simulink model "solar_thermal_control"  (R2024a)
settings: Solver=VariableStepAuto  StartTime=0.0  StopTime=3600*24  FixedStep=0.01  RelTol=1e-3
libraries: fl_lib x41, nesl_utility x20, SimscapeFluids_lib x1
settings Model: Creator=fanzh  LastModifiedBy=fanzh

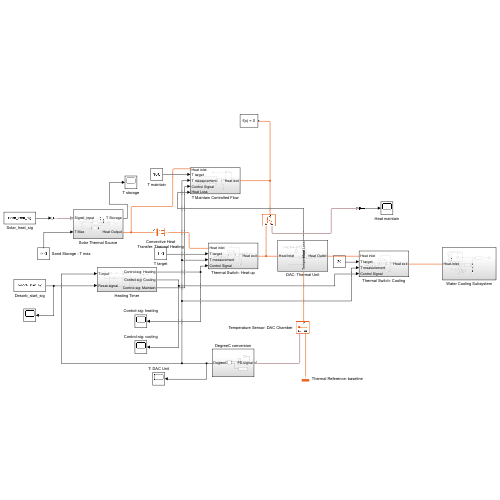
[thumbnail: Simulink's stored preview of the top-level diagram]
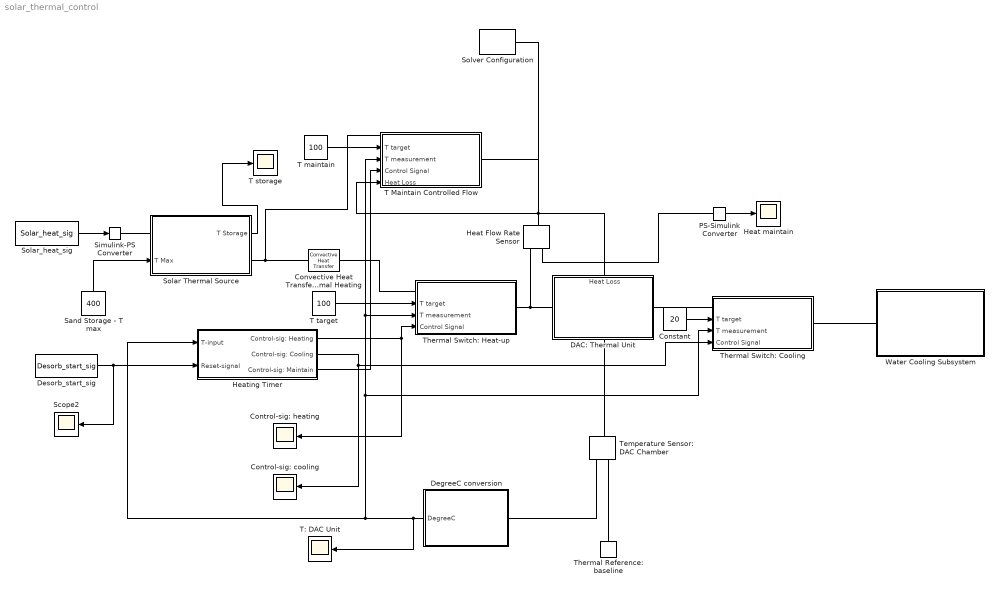
== system solar_thermal_control ==
  Constant : Constant  Value=20
  Control-sig: cooling : Scope
  Control-sig: heating : Scope
  Convective Heat Transfer: Thermal Heating : fl_lib/Thermal/Thermal Elements/Convective Heat Transfer  thermal_type=foundation.enum.constant_variable.constant  area=0.1 m^2  heat_tr_coeff=150 W/(K*m^2)  min_heat_tr_coeff=1e-3 W/(K*m^2)  T_specify=off  T_priority=None  T=0 K  T_nominal_specify=off  T_nominal_value=1  T_nominal_unit=K  Q_specify=off  Q_priority=None  Q=0 W  Q_nominal_specify=off  Q_nominal_value=1  Q_nominal_unit=W
  DAC: Thermal Unit : Subsystem
      settings: PortSchema="{\"entries\":[{\"content\":{\"sides\":[{\"content\":{\"connectorIds\":[\"LConn1\"]},\"type\":\"ConnectorPlacement.EquallySpacedRectSide\",\"uuid\":\"21b9ae42-c24c-4450-b3a3-af5fe19a1042\"},{\"content\":{\"connectorIds\":[\"RConn1\"],\"side\":\"RIGHT\"},\"type\":\"ConnectorPlacement.EquallySpacedRectSide\",\"uuid\":\"0b7693d4-30f7-45cc-b119-858b172421da\"},{\"content\":{\"connectorIds\":[\"Out1\"],\"side\":\"TOP\"},\"type\":\"ConnectorPlacement.EquallySpacedRectSide\",\"uuid\":\"dc3a2d3c-c181-42f7-acd1-46fa5c20e34e\"},{\"content\":{\"connectorIds\":[\"RConn2\"],\"side\":\"BOTTOM\"},\"type\":\"ConnectorPlacement.EquallySpacedRectSide\",\"uuid\":\"1fa3cf11-aa97-4b08-a978-f3583bb285c7\"}]},\"type\":\"ConnectorPlacement.EquallySpacedConnector\",\"uuid\":\"5312b09c-b763-4a63-a4e3-3dc47fafb726\"}],\"packageUris\":[\"http://schema.mathworks.com/mf0/Connector/R2020b\"],\"version\":\"1.0\"}"
  DegreeC conversion : Subsystem
  Desorb_start_sig : FromWorkspace  VariableName=Desorb_start_sig  OutDataTypeStr=boolean  SampleTime=10  Interpolate=off  ZeroCross=off  OutputAfterFinalValue=Holding final value
  Heat Flow Rate Sensor : fl_lib/Thermal/Thermal Sensors/Heat Flow Rate Sensor
  Heat maintain : Scope
  Heating Timer : Subsystem
  PS-Simulink Converter : nesl_utility/PS-Simulink Converter  PhysicalDomain=network_engine_domain  SubClassName=ps_output  LeftPortType=input  RightPortType=output  PseudoPeriodic=off  Frequencies=[]  VectorFormat=inherit  Unit=inherit  AffineConversion=off
  Sand Storage - T max : Constant  Value=400
  Scope2 : Scope
  Simulink-PS Converter : nesl_utility/Simulink-PS Converter  PhysicalDomain=network_engine_domain  SubClassName=ps_input  LeftPortType=input  RightPortType=output  PseudoPeriodic=off  Frequencies=[]  NoiseDistribution=none  NoiseParameters=[]  Unit=J/s  AffineConversion=off  FilteringAndDerivatives=provide  SimscapeFilterOrder=1  InputFilterTimeConstant=0.001  UdotUserProvided=0
  Solar Thermal Source : Subsystem
      settings: PortSchema="{\"entries\":[{\"content\":{\"sides\":[{\"content\":{\"connectorIds\":[\"LConn1\",\"In1\"]},\"type\":\"ConnectorPlacement.EquallySpacedRectSide\",\"uuid\":\"f69a8d61-d6b7-4c5f-bee5-6777f6738a93\"},{\"content\":{\"connectorIds\":[\"Out1\",\"RConn1\"],\"side\":\"RIGHT\"},\"type\":\"ConnectorPlacement.EquallySpacedRectSide\",\"uuid\":\"2abf6aad-3ae7-4bac-8cd7-a5726210c2fc\"},{\"content\":{\"side\":\"TOP\"},\"type\":\"ConnectorPlacement.EquallySpacedRectSide\",\"uuid\":\"e643bfa7-5cdc-456c-a6d6-e9bc07f127d5\"}]},\"type\":\"ConnectorPlacement.EquallySpacedConnector\",\"uuid\":\"a763efd1-4c7b-49c2-88ea-f9b1ada0c58b\"}],\"packageUris\":[\"http://schema.mathworks.com/mf0/Connector/R2020b\"],\"version\":\"1.0\"}"
  Solar_heat_sig : FromWorkspace  VariableName=Solar_heat_sig  SampleTime=10  Interpolate=off  ZeroCross=off  OutputAfterFinalValue=Holding final value
  Solver Configuration : nesl_utility/Solver Configuration  PhysicalDomain=network_engine_domain  SubClassName=solver  LeftPortType=input  RightPortType=generic  Tones=[]  Harmonics=[]  SimulateNoise=off  Profile=off  UseLocalSampling=off  EnableSwitchedLinearOptims=on  FrequencyDomain=off  UseCCode=off  RelTol=0.001  AbsTol=0.001  MinStep=1e-09  ToWorkspace=off  RevertToSquareIcSolve=off  NumHomotopyIterations=100  PhasorMode=off  PhasorModeNumHarmonics=1  ConsistencySolver=NEWTON_XTOL_AFTER_FTOL  IndexReductionMethod=DerivativeReplacement  DoDC=off  ResidualTolerance=1e-09  ConsistencyTolSource=GLOBAL  ConsistencyAbsTol=0.001  ConsistencyRelTol=0.001  ConsistencyTolFactor=0.001  UseLocalSolver=off  LocalSolverChoice=NE_BACKWARD_EULER_ADVANCER  ResolveIndetEquations=on  FunctionEvalNumThread=1  LocalSolverSampleTime=0.001  DoFixedCost=off  MaxNonlinIter=3  MaxModeIter=2  ComputeImpulses=off  ImpulseIterations=2  LinearAlgebra=auto  LinearAlgebraNumThread=0  EquationFormulation=NE_TIME_EF  DelaysMemoryBudget=1024  AutomaticFiltering=on  FilteringTimeConstant=0.001  PartitionStorageMethod=AS_NEEDED  PartitionMemoryBudget=1024  PartitionMethod=ROBUST  MultibodyUseLocalSolver=off  MultibodyLocalSolverChoice=ODE1  MultibodyLocalSolverSampleTime=0.001
  T Maintain Controlled Flow : Subsystem
      settings: PortSchema="{\"entries\":[{\"content\":{\"sides\":[{\"content\":{\"connectorIds\":[\"LConn1\",\"In1\",\"In2\",\"In3\",\"In4\"]},\"type\":\"ConnectorPlacement.EquallySpacedRectSide\",\"uuid\":\"eab90983-c678-4d00-88f4-d7eb0332fabb\"},{\"content\":{\"connectorIds\":[\"RConn1\"],\"side\":\"RIGHT\"},\"type\":\"ConnectorPlacement.EquallySpacedRectSide\",\"uuid\":\"4911cae5-9d9f-472e-86e2-92bac9c7b6a6\"},{\"content\":{\"side\":\"TOP\"},\"type\":\"ConnectorPlacement.EquallySpacedRectSide\",\"uuid\":\"e0869e9b-2d53-4209-96a5-637bff90aadc\"}]},\"type\":\"ConnectorPlacement.EquallySpacedConnector\",\"uuid\":\"c03f20a9-89c5-4bd4-ab09-4122887b8deb\"}],\"packageUris\":[\"http://schema.mathworks.com/mf0/Connector/R2020b\"],\"version\":\"1.0\"}"
  T maintain : Constant  Value=100
  T storage : Scope
  T target : Constant  Value=100
  T: DAC Unit : Scope
  "Temperature Sensor: DAC Chamber " : fl_lib/Thermal/Thermal Sensors/Temperature Sensor  temperature_measure=foundation.enum.MeasurementReference.difference
  Thermal Reference: baseline : fl_lib/Thermal/Thermal Elements/Thermal Reference
  Thermal Switch: Cooling : Subsystem
      settings: PortSchema="{\"entries\":[{\"content\":{\"sides\":[{\"content\":{\"connectorIds\":[\"LConn1\",\"In1\",\"In2\",\"In3\"]},\"type\":\"ConnectorPlacement.EquallySpacedRectSide\",\"uuid\":\"eab90983-c678-4d00-88f4-d7eb0332fabb\"},{\"content\":{\"connectorIds\":[\"RConn1\"],\"side\":\"RIGHT\"},\"type\":\"ConnectorPlacement.EquallySpacedRectSide\",\"uuid\":\"4911cae5-9d9f-472e-86e2-92bac9c7b6a6\"},{\"content\":{\"side\":\"TOP\"},\"type\":\"ConnectorPlacement.EquallySpacedRectSide\",\"uuid\":\"e0869e9b-2d53-4209-96a5-637bff90aadc\"}]},\"type\":\"ConnectorPlacement.EquallySpacedConnector\",\"uuid\":\"c03f20a9-89c5-4bd4-ab09-4122887b8deb\"}],\"packageUris\":[\"http://schema.mathworks.com/mf0/Connector/R2020b\"],\"version\":\"1.0\"}"
  Thermal Switch: Heat-up : Subsystem
      settings: PortSchema="{\"entries\":[{\"content\":{\"sides\":[{\"content\":{\"connectorIds\":[\"LConn1\",\"In1\",\"In2\",\"In3\"]},\"type\":\"ConnectorPlacement.EquallySpacedRectSide\",\"uuid\":\"eab90983-c678-4d00-88f4-d7eb0332fabb\"},{\"content\":{\"connectorIds\":[\"RConn1\"],\"side\":\"RIGHT\"},\"type\":\"ConnectorPlacement.EquallySpacedRectSide\",\"uuid\":\"4911cae5-9d9f-472e-86e2-92bac9c7b6a6\"},{\"content\":{\"side\":\"TOP\"},\"type\":\"ConnectorPlacement.EquallySpacedRectSide\",\"uuid\":\"e0869e9b-2d53-4209-96a5-637bff90aadc\"}]},\"type\":\"ConnectorPlacement.EquallySpacedConnector\",\"uuid\":\"c03f20a9-89c5-4bd4-ab09-4122887b8deb\"}],\"packageUris\":[\"http://schema.mathworks.com/mf0/Connector/R2020b\"],\"version\":\"1.0\"}"
  Water Cooling Subsystem : Subsystem
  wires:
  T target/1 -> Thermal Switch: Heat-up/1(T target)
  Constant/1 -> Thermal Switch: Cooling/1(T target)
  Heating Timer/1(Control-sig: Heating) -> Control-sig: heating/1, Thermal Switch: Heat-up/3(Control Signal)
  Heating Timer/2(Control-sig: Cooling) -> Control-sig: cooling/1, Thermal Switch: Cooling/3(Control Signal)
  Solar_heat_sig/1 -> Simulink-PS Converter/1
  Sand Storage - T max/1 -> Solar Thermal Source/1(T Max)
  Desorb_start_sig/1 -> Heating Timer/2(Reset-signal), Scope2/1
  T maintain/1 -> T Maintain Controlled Flow/1(T target)
  PS-Simulink Converter/1 -> Heat maintain/1
  Heating Timer/3(Control-sig: Maintain) -> T Maintain Controlled Flow/3(Control Signal)
  DegreeC conversion/1(DegreeC) -> Thermal Switch: Cooling/2(T measurement), Thermal Switch: Heat-up/2(T measurement), T Maintain Controlled Flow/2(T measurement), Heating Timer/1(T-input), T: DAC Unit/1
  Solar Thermal Source/1(T Storage) -> T storage/1
  DAC: Thermal Unit/1(Heat Loss) -> T Maintain Controlled Flow/4(Heat Loss)
  connections:
  "Temperature Sensor: DAC Chamber "/RConn1 -- Thermal Reference: baseline/LConn1
  Thermal Switch: Heat-up/RConn1 -- Heat Flow Rate Sensor/RConn2 -- DAC: Thermal Unit/LConn1
  Thermal Switch: Heat-up/LConn1 -- Convective Heat Transfer: Thermal Heating/RConn1
  "Temperature Sensor: DAC Chamber "/LConn1 -- DAC: Thermal Unit/RConn2
  "Temperature Sensor: DAC Chamber "/RConn2 -- DegreeC conversion/LConn1
  DAC: Thermal Unit/RConn1 -- Thermal Switch: Cooling/LConn1
  Water Cooling Subsystem/LConn1 -- Thermal Switch: Cooling/RConn1
  Simulink-PS Converter/RConn1 -- Solar Thermal Source/LConn1
  PS-Simulink Converter/LConn1 -- Heat Flow Rate Sensor/RConn1
  Heat Flow Rate Sensor/LConn1 -- T Maintain Controlled Flow/RConn1 -- Solver Configuration/RConn1
  Convective Heat Transfer: Thermal Heating/LConn1 -- T Maintain Controlled Flow/LConn1 -- Solar Thermal Source/RConn1

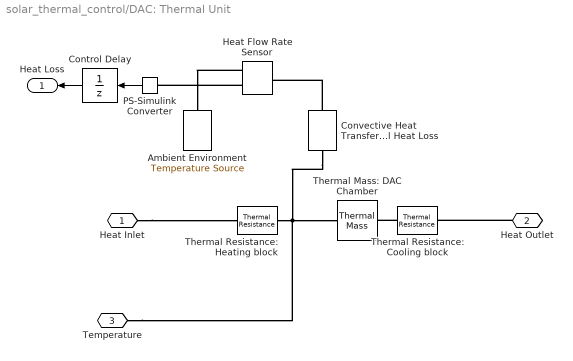
== system solar_thermal_control/DAC: Thermal Unit ==
  Ambient Environment : fl_lib/Thermal/Thermal Sources/Temperature Source  temperature=15 degC
  Control Delay : UnitDelay  SampleTime=-1  HasFrameUpgradeWarning=on
  Convective Heat Transfer: Natural Heat Loss : fl_lib/Thermal/Thermal Elements/Convective Heat Transfer  thermal_type=foundation.enum.constant_variable.constant  area=0.05 m^2  heat_tr_coeff=4 W/(K*m^2)  min_heat_tr_coeff=1e-3 W/(K*m^2)  T_specify=off  T_priority=None  T=0 K  T_nominal_specify=off  T_nominal_value=1  T_nominal_unit=K  Q_specify=off  Q_priority=None  Q=0 W  Q_nominal_specify=off  Q_nominal_value=1  Q_nominal_unit=W
  Heat Flow Rate Sensor : fl_lib/Thermal/Thermal Sensors/Heat Flow Rate Sensor
  PS-Simulink Converter : nesl_utility/PS-Simulink Converter  PhysicalDomain=network_engine_domain  SubClassName=ps_output  LeftPortType=input  RightPortType=output  PseudoPeriodic=off  Frequencies=[]  VectorFormat=inherit  Unit=inherit  AffineConversion=off
  Thermal Mass: DAC Chamber : fl_lib/Thermal/Thermal Elements/Thermal Mass  mass_type=foundation.enum.constant_variable.constant  mass=2 kg  sp_heat=447 J/(K*kg)  mass_min=1e-6 kg  num_ports=foundation.enum.numPorts2.two  m_specify=off  m_priority=High  m=1 kg  m_nominal_specify=off  m_nominal_value=1  m_nominal_unit=kg  T_specify=on  T_priority=High  T=15 degC  T_nominal_specify=off  T_nominal_value=1  T_nominal_unit=K  Q_specify=off  Q_priority=None  Q=0 W  Q_nominal_specify=off  Q_nominal_value=1  Q_nominal_unit=W
      settings: InternalSimscapePortConfiguration="{\"Bottom\":[],\"Left\":[{\"id\":\"M\",\"label\":\"\",\"type\":\"foundation.thermal.thermal\"}],\"Right\":[{\"id\":\"N\",\"label\":\"\",\"type\":\"foundation.thermal.thermal\"}],\"Top\":[]}"
  Thermal Resistance: Cooling block : fl_lib/Thermal/Thermal Elements/Thermal Resistance  resistance=0.1 K/W  T_specify=off  T_priority=None  T=0 K  T_nominal_specify=off  T_nominal_value=1  T_nominal_unit=K  Q_specify=off  Q_priority=None  Q=0 W  Q_nominal_specify=off  Q_nominal_value=1  Q_nominal_unit=W
  Thermal Resistance: Heating block : fl_lib/Thermal/Thermal Elements/Thermal Resistance  resistance=1 K/W  T_specify=off  T_priority=None  T=0 K  T_nominal_specify=off  T_nominal_value=1  T_nominal_unit=K  Q_specify=off  Q_priority=None  Q=0 W  Q_nominal_specify=off  Q_nominal_value=1  Q_nominal_unit=W
  Heat Inlet : PMIOPort  Side=Left
  Heat Outlet : PMIOPort  Port=2  Side=Right
  Temperature : PMIOPort  Port=3  Side=Right
  Heat Loss : Outport
  wires:
  PS-Simulink Converter/1 -> Control Delay/1
  Control Delay/1 -> Heat Loss/1
  connections:
  Heat Inlet/RConn1 -- Thermal Resistance: Heating block/LConn1
  Thermal Resistance: Heating block/RConn1 -- Thermal Mass: DAC Chamber/LConn1 -- Convective Heat Transfer: Natural Heat Loss/LConn1 -- Temperature/RConn1
  Thermal Resistance: Cooling block/LConn1 -- Thermal Mass: DAC Chamber/RConn1
  Heat Outlet/RConn1 -- Thermal Resistance: Cooling block/RConn1
  Convective Heat Transfer: Natural Heat Loss/RConn1 -- Heat Flow Rate Sensor/LConn1
  Heat Flow Rate Sensor/RConn2 -- Ambient Environment/LConn1
  Heat Flow Rate Sensor/RConn1 -- PS-Simulink Converter/LConn1

== system solar_thermal_control/DegreeC conversion ==
  Absolute zero reference : Constant  Value=-273.15
  PS-Simulink Converter : nesl_utility/PS-Simulink Converter  PhysicalDomain=network_engine_domain  SubClassName=ps_output  LeftPortType=input  RightPortType=output  PseudoPeriodic=off  Frequencies=[]  VectorFormat=inherit  Unit=inherit  AffineConversion=off
  T: degreeC : Sum
  PS-signal : PMIOPort  Side=Left
  DegreeC : Outport
  wires:
  Absolute zero reference/1 -> T: degreeC/2
  PS-Simulink Converter/1 -> T: degreeC/1
  T: degreeC/1 -> DegreeC/1
  connections:
  PS-signal/RConn1 -- PS-Simulink Converter/LConn1

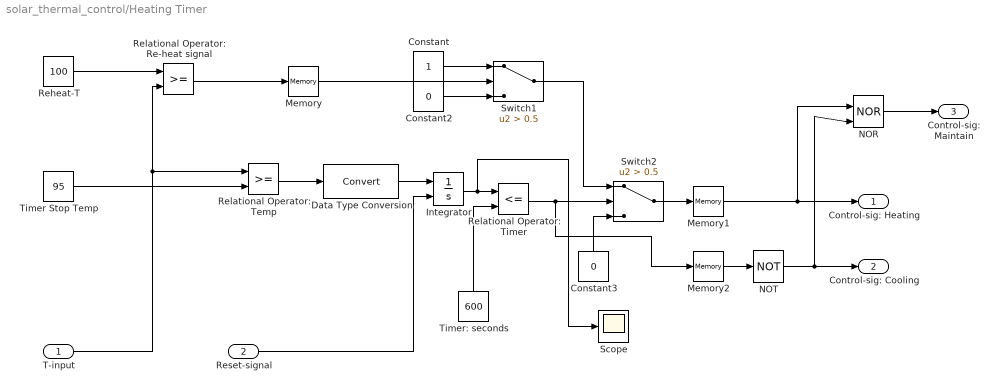
== system solar_thermal_control/Heating Timer ==
  T-input : Inport
  Reset-signal : Inport  Port=2
  Constant : Constant
  Constant2 : Constant  Value=0
  Constant3 : Constant  Value=0
  Data Type Conversion : DataTypeConversion  SaturateOnIntegerOverflow=off  RndMeth=Floor
  Integrator : Integrator  ExternalReset=level hold
  Memory : Memory
  Memory1 : Memory
  Memory2 : Memory
  NOR : Logic  Operator=NOR  IconShape=distinctive  AllPortsSameDT=off  OutDataTypeStr=boolean
  NOT : Logic  Operator=NOT  IconShape=distinctive  AllPortsSameDT=off  OutDataTypeStr=boolean
  Reheat-T : Constant  Value=100
  Relational Operator: Re-heat signal : RelationalOperator  OutDataTypeStr=boolean  RndMeth=Simplest  InputSameDT=off
  Relational Operator: Temp : RelationalOperator  OutDataTypeStr=boolean  RndMeth=Simplest  InputSameDT=off
  Relational Operator: Timer : RelationalOperator  Operator=<=  OutDataTypeStr=boolean  RndMeth=Simplest  InputSameDT=off
  Scope : Scope
  Switch1 : Switch  Criteria=u2 > Threshold  Threshold=0.5  SaturateOnIntegerOverflow=off  InputSameDT=off
  Switch2 : Switch  Criteria=u2 > Threshold  Threshold=0.5  SaturateOnIntegerOverflow=off  InputSameDT=off
  Timer Stop Temp : Constant  Value=95
  Timer: seconds : Constant  Value=600
  Control-sig: Heating : Outport
  Control-sig: Cooling : Outport  Port=2
  Control-sig: Maintain : Outport  Port=3
  wires:
  Relational Operator: Temp/1 -> Data Type Conversion/1
  T-input/1 -> Relational Operator: Re-heat signal/2, Relational Operator: Temp/1
  Data Type Conversion/1 -> Integrator/1
  Timer Stop Temp/1 -> Relational Operator: Temp/2
  Timer: seconds/1 -> Relational Operator: Timer/2
  Constant/1 -> Switch1/1
  Switch1/1 -> Switch2/1
  Constant2/1 -> Switch1/3
  Constant3/1 -> Switch2/3
  Switch2/1 -> Memory1/1
  Relational Operator: Re-heat signal/1 -> Memory/1
  Memory/1 -> Switch1/2
  Memory1/1 -> NOR/1, Control-sig: Heating/1
  Integrator/1 -> Scope/1, Relational Operator: Timer/1
  Reset-signal/1 -> Integrator/2
  Relational Operator: Timer/1 -> Memory2/1, Switch2/2
  Memory2/1 -> NOT/1
  Reheat-T/1 -> Relational Operator: Re-heat signal/1
  NOT/1 -> NOR/2, Control-sig: Cooling/1
  NOR/1 -> Control-sig: Maintain/1

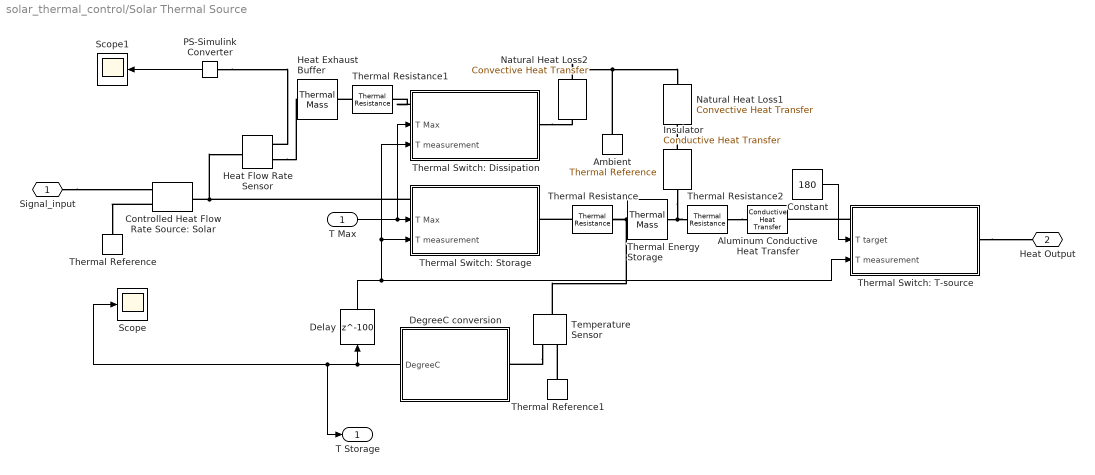
== system solar_thermal_control/Solar Thermal Source ==
  T Max : Inport
  Aluminum Conductive Heat Transfer : fl_lib/Thermal/Thermal Elements/Conductive Heat Transfer  thermal_type=foundation.enum.ConstantVariableTabulated.Constant  wall_geometry=foundation.enum.ConductionWallGeometry.Planar  area=4e-3 m^2  thickness=0.1 m  d_in=0.05 m  d_out=0.1 m  L=1 m  th_cond_min=10 W/(K*m)  th_cond=237 W/(K*m)  th_cond_TLU=[413, 401, 392, 383, 371, 357, 342] W/(K*m)  temp_TLU=[200, 273, 400, 600, 800, 1000, 1200] K  T_specify=off  T_priority=None  T=0 K  T_nominal_specify=off  T_nominal_value=1  T_nominal_unit=K  Q_specify=off  Q_priority=None  Q=0 W  Q_nominal_specify=off  Q_nominal_value=1  Q_nominal_unit=W
  Ambient : fl_lib/Thermal/Thermal Elements/Thermal Reference
  Constant : Constant  Value=180
  Controlled Heat Flow Rate Source: Solar : fl_lib/Thermal/Thermal Sources/Controlled Heat Flow Rate Source
  DegreeC conversion : Subsystem
  Delay : Delay  DelayLength=100  InitialCondition=0
  Heat Exhaust Buffer : fl_lib/Thermal/Thermal Elements/Thermal Mass  mass_type=foundation.enum.constant_variable.constant  mass=0.5 kg  sp_heat=840 J/(K*kg)  mass_min=1e-6 kg  num_ports=foundation.enum.numPorts2.two  m_specify=off  m_priority=High  m=1 kg  m_nominal_specify=off  m_nominal_value=1  m_nominal_unit=kg  T_specify=on  T_priority=High  T=400 K  T_nominal_specify=off  T_nominal_value=1  T_nominal_unit=K  Q_specify=off  Q_priority=None  Q=0 W  Q_nominal_specify=off  Q_nominal_value=1  Q_nominal_unit=W
      settings: InternalSimscapePortConfiguration="{\"Bottom\":[],\"Left\":[{\"id\":\"M\",\"label\":\"\",\"type\":\"foundation.thermal.thermal\"}],\"Right\":[{\"id\":\"N\",\"label\":\"\",\"type\":\"foundation.thermal.thermal\"}],\"Top\":[]}"
  Heat Flow Rate Sensor : fl_lib/Thermal/Thermal Sensors/Heat Flow Rate Sensor
  Insulator : fl_lib/Thermal/Thermal Elements/Conductive Heat Transfer  thermal_type=foundation.enum.ConstantVariableTabulated.Constant  wall_geometry=foundation.enum.ConductionWallGeometry.Planar  area=1e-3 m^2  thickness=0.1 m  d_in=0.05 m  d_out=0.1 m  L=1 m  th_cond_min=10 W/(K*m)  th_cond=0.1 W/(K*m)  th_cond_TLU=[413, 401, 392, 383, 371, 357, 342] W/(K*m)  temp_TLU=[200, 273, 400, 600, 800, 1000, 1200] K  T_specify=off  T_priority=None  T=0 K  T_nominal_specify=off  T_nominal_value=1  T_nominal_unit=K  Q_specify=off  Q_priority=None  Q=0 W  Q_nominal_specify=off  Q_nominal_value=1  Q_nominal_unit=W
  Natural Heat Loss1 : fl_lib/Thermal/Thermal Elements/Convective Heat Transfer  thermal_type=foundation.enum.constant_variable.constant  area=1e-3 m^2  heat_tr_coeff=10 W/(K*m^2)  min_heat_tr_coeff=1e-3 W/(K*m^2)  T_specify=off  T_priority=None  T=0 K  T_nominal_specify=off  T_nominal_value=1  T_nominal_unit=K  Q_specify=off  Q_priority=None  Q=0 W  Q_nominal_specify=off  Q_nominal_value=1  Q_nominal_unit=W
  Natural Heat Loss2 : fl_lib/Thermal/Thermal Elements/Convective Heat Transfer  thermal_type=foundation.enum.constant_variable.constant  area=1 m^2  heat_tr_coeff=10 W/(K*m^2)  min_heat_tr_coeff=1e-3 W/(K*m^2)  T_specify=off  T_priority=None  T=0 K  T_nominal_specify=off  T_nominal_value=1  T_nominal_unit=K  Q_specify=off  Q_priority=None  Q=0 W  Q_nominal_specify=off  Q_nominal_value=1  Q_nominal_unit=W
  PS-Simulink Converter : nesl_utility/PS-Simulink Converter  PhysicalDomain=network_engine_domain  SubClassName=ps_output  LeftPortType=input  RightPortType=output  PseudoPeriodic=off  Frequencies=[]  VectorFormat=inherit  Unit=inherit  AffineConversion=off
  Scope : Scope
  Scope1 : Scope
  Temperature Sensor : fl_lib/Thermal/Thermal Sensors/Temperature Sensor  temperature_measure=foundation.enum.MeasurementReference.difference
  Thermal Energy Storage : fl_lib/Thermal/Thermal Elements/Thermal Mass  mass_type=foundation.enum.constant_variable.constant  mass=5 kg  sp_heat=840 J/(K*kg)  mass_min=1e-6 kg  num_ports=foundation.enum.numPorts2.two  m_specify=off  m_priority=High  m=1 kg  m_nominal_specify=off  m_nominal_value=1  m_nominal_unit=kg  T_specify=on  T_priority=High  T=400 K  T_nominal_specify=off  T_nominal_value=1  T_nominal_unit=K  Q_specify=off  Q_priority=None  Q=0 W  Q_nominal_specify=off  Q_nominal_value=1  Q_nominal_unit=W
      settings: InternalSimscapePortConfiguration="{\"Bottom\":[],\"Left\":[{\"id\":\"M\",\"label\":\"\",\"type\":\"foundation.thermal.thermal\"}],\"Right\":[{\"id\":\"N\",\"label\":\"\",\"type\":\"foundation.thermal.thermal\"}],\"Top\":[]}"
  Thermal Reference : fl_lib/Thermal/Thermal Elements/Thermal Reference
  Thermal Reference1 : fl_lib/Thermal/Thermal Elements/Thermal Reference
  Thermal Resistance : fl_lib/Thermal/Thermal Elements/Thermal Resistance  resistance=10 K/W  T_specify=off  T_priority=None  T=0 K  T_nominal_specify=off  T_nominal_value=1  T_nominal_unit=K  Q_specify=off  Q_priority=None  Q=0 W  Q_nominal_specify=off  Q_nominal_value=1  Q_nominal_unit=W
  Thermal Resistance1 : fl_lib/Thermal/Thermal Elements/Thermal Resistance  resistance=10 K/W  T_specify=off  T_priority=None  T=0 K  T_nominal_specify=off  T_nominal_value=1  T_nominal_unit=K  Q_specify=off  Q_priority=None  Q=0 W  Q_nominal_specify=off  Q_nominal_value=1  Q_nominal_unit=W
  Thermal Resistance2 : fl_lib/Thermal/Thermal Elements/Thermal Resistance  resistance=1 K/W  T_specify=off  T_priority=None  T=0 K  T_nominal_specify=off  T_nominal_value=1  T_nominal_unit=K  Q_specify=off  Q_priority=None  Q=0 W  Q_nominal_specify=off  Q_nominal_value=1  Q_nominal_unit=W
  Thermal Switch: Dissipation : Subsystem
      settings: PortSchema="{\"entries\":[{\"content\":{\"sides\":[{\"content\":{\"connectorIds\":[\"LConn1\",\"In1\",\"In2\"]},\"type\":\"ConnectorPlacement.EquallySpacedRectSide\",\"uuid\":\"eab90983-c678-4d00-88f4-d7eb0332fabb\"},{\"content\":{\"connectorIds\":[\"RConn1\"],\"side\":\"RIGHT\"},\"type\":\"ConnectorPlacement.EquallySpacedRectSide\",\"uuid\":\"4911cae5-9d9f-472e-86e2-92bac9c7b6a6\"},{\"content\":{\"side\":\"TOP\"},\"type\":\"ConnectorPlacement.EquallySpacedRectSide\",\"uuid\":\"e0869e9b-2d53-4209-96a5-637bff90aadc\"}]},\"type\":\"ConnectorPlacement.EquallySpacedConnector\",\"uuid\":\"c03f20a9-89c5-4bd4-ab09-4122887b8deb\"}],\"packageUris\":[\"http://schema.mathworks.com/mf0/Connector/R2020b\"],\"version\":\"1.0\"}"
  Thermal Switch: Storage : Subsystem
      settings: PortSchema="{\"entries\":[{\"content\":{\"sides\":[{\"content\":{\"connectorIds\":[\"LConn1\",\"In1\",\"In2\"]},\"type\":\"ConnectorPlacement.EquallySpacedRectSide\",\"uuid\":\"eab90983-c678-4d00-88f4-d7eb0332fabb\"},{\"content\":{\"connectorIds\":[\"RConn1\"],\"side\":\"RIGHT\"},\"type\":\"ConnectorPlacement.EquallySpacedRectSide\",\"uuid\":\"4911cae5-9d9f-472e-86e2-92bac9c7b6a6\"},{\"content\":{\"side\":\"TOP\"},\"type\":\"ConnectorPlacement.EquallySpacedRectSide\",\"uuid\":\"e0869e9b-2d53-4209-96a5-637bff90aadc\"}]},\"type\":\"ConnectorPlacement.EquallySpacedConnector\",\"uuid\":\"c03f20a9-89c5-4bd4-ab09-4122887b8deb\"}],\"packageUris\":[\"http://schema.mathworks.com/mf0/Connector/R2020b\"],\"version\":\"1.0\"}"
  Thermal Switch: T-source : Subsystem
      settings: PortSchema="{\"entries\":[{\"content\":{\"sides\":[{\"content\":{\"connectorIds\":[\"LConn1\",\"In1\",\"In2\"]},\"type\":\"ConnectorPlacement.EquallySpacedRectSide\",\"uuid\":\"eab90983-c678-4d00-88f4-d7eb0332fabb\"},{\"content\":{\"connectorIds\":[\"RConn1\"],\"side\":\"RIGHT\"},\"type\":\"ConnectorPlacement.EquallySpacedRectSide\",\"uuid\":\"4911cae5-9d9f-472e-86e2-92bac9c7b6a6\"},{\"content\":{\"side\":\"TOP\"},\"type\":\"ConnectorPlacement.EquallySpacedRectSide\",\"uuid\":\"e0869e9b-2d53-4209-96a5-637bff90aadc\"}]},\"type\":\"ConnectorPlacement.EquallySpacedConnector\",\"uuid\":\"c03f20a9-89c5-4bd4-ab09-4122887b8deb\"}],\"packageUris\":[\"http://schema.mathworks.com/mf0/Connector/R2020b\"],\"version\":\"1.0\"}"
  Signal_input : PMIOPort  Side=Left
  Heat Output : PMIOPort  Port=2  Side=Right
  T Storage : Outport
  wires:
  T Max/1 -> Thermal Switch: Dissipation/1(T Max), Thermal Switch: Storage/1(T Max)
  DegreeC conversion/1(DegreeC) -> T Storage/1, Scope/1, Delay/1
  PS-Simulink Converter/1 -> Scope1/1
  Constant/1 -> Thermal Switch: T-source/1(T target)
  Delay/1 -> Thermal Switch: Storage/2(T measurement), Thermal Switch: Dissipation/2(T measurement), Thermal Switch: T-source/2(T measurement)
  connections:
  Ambient/LConn1 -- Natural Heat Loss2/RConn1 -- Natural Heat Loss1/RConn1
  Thermal Energy Storage/LConn1 -- Insulator/LConn1 -- Thermal Resistance2/LConn1
  Thermal Energy Storage/RConn1 -- Temperature Sensor/LConn1 -- Thermal Resistance/RConn1
  Temperature Sensor/RConn2 -- DegreeC conversion/LConn1
  Thermal Reference1/LConn1 -- Temperature Sensor/RConn1
  Insulator/RConn1 -- Natural Heat Loss1/LConn1
  Controlled Heat Flow Rate Source: Solar/RConn2 -- Thermal Reference/LConn1
  Signal_input/RConn1 -- Controlled Heat Flow Rate Source: Solar/RConn1
  Thermal Switch: Dissipation/RConn1 -- Natural Heat Loss2/LConn1
  PS-Simulink Converter/LConn1 -- Heat Flow Rate Sensor/RConn1
  Thermal Resistance/LConn1 -- Thermal Switch: Storage/RConn1
  Thermal Switch: Storage/LConn1 -- Heat Flow Rate Sensor/LConn1 -- Controlled Heat Flow Rate Source: Solar/LConn1
  Thermal Switch: T-source/LConn1 -- Aluminum Conductive Heat Transfer/RConn1
  Thermal Switch: T-source/RConn1 -- Heat Output/RConn1
  Heat Flow Rate Sensor/RConn2 -- Heat Exhaust Buffer/RConn1
  Thermal Resistance1/LConn1 -- Heat Exhaust Buffer/LConn1
  Thermal Switch: Dissipation/LConn1 -- Thermal Resistance1/RConn1
  Thermal Resistance2/RConn1 -- Aluminum Conductive Heat Transfer/LConn1

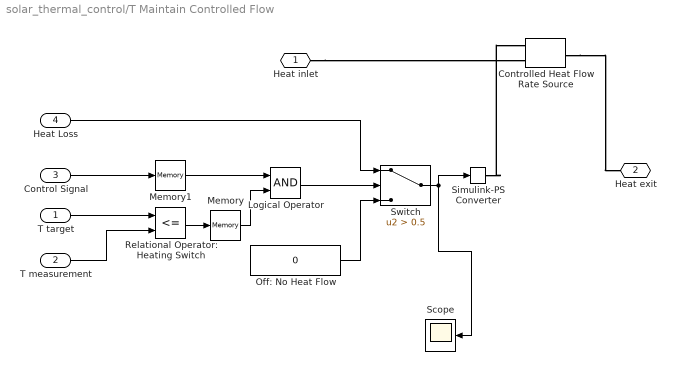
== system solar_thermal_control/T Maintain Controlled Flow ==
  T target : Inport
  T measurement : Inport  Port=2
  Control Signal : Inport  Port=3
  Heat Loss : Inport  Port=4
  Controlled Heat Flow Rate Source : fl_lib/Thermal/Thermal Sources/Controlled Heat Flow Rate Source
  Logical Operator : Logic  AllPortsSameDT=off  OutDataTypeStr=boolean
  Memory : Memory
  Memory1 : Memory
  Off: No Heat Flow : Constant  Value=0
  Relational Operator: Heating Switch : RelationalOperator  Operator=<=  OutDataTypeStr=boolean  RndMeth=Simplest  InputSameDT=off
  Scope : Scope
  Simulink-PS Converter : nesl_utility/Simulink-PS Converter  PhysicalDomain=network_engine_domain  SubClassName=ps_input  LeftPortType=input  RightPortType=output  PseudoPeriodic=off  Frequencies=[]  NoiseDistribution=none  NoiseParameters=[]  Unit=1  AffineConversion=off  FilteringAndDerivatives=provide  SimscapeFilterOrder=1  InputFilterTimeConstant=0.001  UdotUserProvided=0
  Switch : Switch  Criteria=u2 > Threshold  Threshold=0.5  SaturateOnIntegerOverflow=off  InputSameDT=off
  Heat inlet : PMIOPort  Side=Left
  Heat exit : PMIOPort  Port=2  Side=Right
  wires:
  Relational Operator: Heating Switch/1 -> Memory/1
  T measurement/1 -> Relational Operator: Heating Switch/2
  Off: No Heat Flow/1 -> Switch/3
  Switch/1 -> Scope/1, Simulink-PS Converter/1
  T target/1 -> Relational Operator: Heating Switch/1
  Memory/1 -> Logical Operator/2
  Logical Operator/1 -> Switch/2
  Heat Loss/1 -> Switch/1
  Control Signal/1 -> Memory1/1
  Memory1/1 -> Logical Operator/1
  connections:
  Simulink-PS Converter/RConn1 -- Controlled Heat Flow Rate Source/RConn1
  Controlled Heat Flow Rate Source/LConn1 -- Heat exit/RConn1
  Heat inlet/RConn1 -- Controlled Heat Flow Rate Source/RConn2

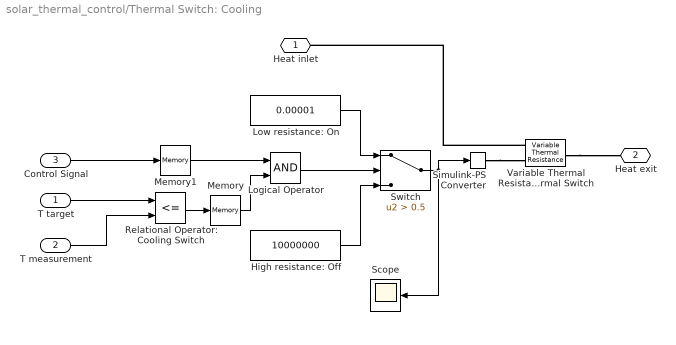
== system solar_thermal_control/Thermal Switch: Cooling ==
  T target : Inport
  T measurement : Inport  Port=2
  Control Signal : Inport  Port=3
  High resistance: Off : Constant  Value=10000000
  Logical Operator : Logic  AllPortsSameDT=off  OutDataTypeStr=boolean
  Low resistance: On : Constant  Value=0.00001
  Memory : Memory
  Memory1 : Memory
  Relational Operator: Cooling Switch : RelationalOperator  Operator=<=  OutDataTypeStr=boolean  RndMeth=Simplest  InputSameDT=off
  Scope : Scope
  Simulink-PS Converter : nesl_utility/Simulink-PS Converter  PhysicalDomain=network_engine_domain  SubClassName=ps_input  LeftPortType=input  RightPortType=output  PseudoPeriodic=off  Frequencies=[]  NoiseDistribution=none  NoiseParameters=[]  Unit=1  AffineConversion=off  FilteringAndDerivatives=provide  SimscapeFilterOrder=1  InputFilterTimeConstant=0.001  UdotUserProvided=0
  Switch : Switch  Criteria=u2 > Threshold  Threshold=0.5  SaturateOnIntegerOverflow=off  InputSameDT=off
  Variable Thermal Resistance: Thermal Switch : fl_lib/Thermal/Thermal Elements/Variable Thermal Resistance  R_min=0 K/W  T_specify=off  T_priority=None  T=0 K  T_nominal_specify=off  T_nominal_value=1  T_nominal_unit=K  Q_specify=off  Q_priority=None  Q=0 W  Q_nominal_specify=off  Q_nominal_value=1  Q_nominal_unit=W
      settings: InternalSimscapePortConfiguration="{\"Bottom\":[],\"Left\":[{\"id\":\"A\",\"label\":\"A\",\"type\":\"foundation.thermal.thermal\"},{\"id\":\"R\",\"label\":\"R\",\"type\":\"input\"}],\"Right\":[{\"id\":\"B\",\"label\":\"B\",\"type\":\"foundation.thermal.thermal\"}],\"Top\":[]}"
  Heat inlet : PMIOPort  Side=Left
  Heat exit : PMIOPort  Port=2  Side=Right
  wires:
  Relational Operator: Cooling Switch/1 -> Memory/1
  T measurement/1 -> Relational Operator: Cooling Switch/2
  High resistance: Off/1 -> Switch/3
  Switch/1 -> Scope/1, Simulink-PS Converter/1
  T target/1 -> Relational Operator: Cooling Switch/1
  Memory/1 -> Logical Operator/2
  Logical Operator/1 -> Switch/2
  Low resistance: On/1 -> Switch/1
  Control Signal/1 -> Memory1/1
  Memory1/1 -> Logical Operator/1
  connections:
  Simulink-PS Converter/RConn1 -- Variable Thermal Resistance: Thermal Switch/LConn2
  Variable Thermal Resistance: Thermal Switch/LConn1 -- Heat inlet/RConn1
  Variable Thermal Resistance: Thermal Switch/RConn1 -- Heat exit/RConn1

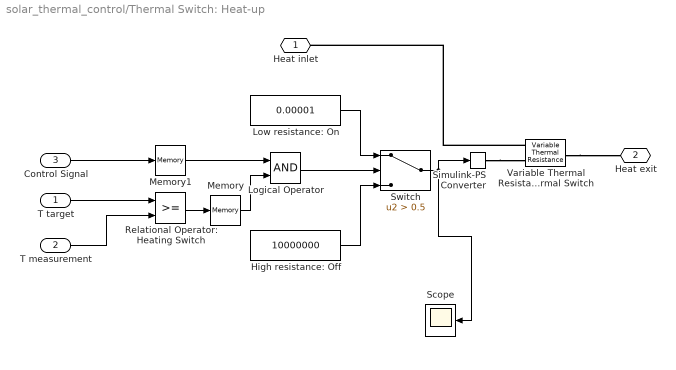
== system solar_thermal_control/Thermal Switch: Heat-up ==
  T target : Inport
  T measurement : Inport  Port=2
  Control Signal : Inport  Port=3
  High resistance: Off : Constant  Value=10000000
  Logical Operator : Logic  AllPortsSameDT=off  OutDataTypeStr=boolean
  Low resistance: On : Constant  Value=0.00001
  Memory : Memory
  Memory1 : Memory
  Relational Operator: Heating Switch : RelationalOperator  OutDataTypeStr=boolean  RndMeth=Simplest  InputSameDT=off
  Scope : Scope
  Simulink-PS Converter : nesl_utility/Simulink-PS Converter  PhysicalDomain=network_engine_domain  SubClassName=ps_input  LeftPortType=input  RightPortType=output  PseudoPeriodic=off  Frequencies=[]  NoiseDistribution=none  NoiseParameters=[]  Unit=1  AffineConversion=off  FilteringAndDerivatives=provide  SimscapeFilterOrder=1  InputFilterTimeConstant=0.001  UdotUserProvided=0
  Switch : Switch  Criteria=u2 > Threshold  Threshold=0.5  SaturateOnIntegerOverflow=off  InputSameDT=off
  Variable Thermal Resistance: Thermal Switch : fl_lib/Thermal/Thermal Elements/Variable Thermal Resistance  R_min=0 K/W  T_specify=off  T_priority=None  T=0 K  T_nominal_specify=off  T_nominal_value=1  T_nominal_unit=K  Q_specify=off  Q_priority=None  Q=0 W  Q_nominal_specify=off  Q_nominal_value=1  Q_nominal_unit=W
      settings: InternalSimscapePortConfiguration="{\"Bottom\":[],\"Left\":[{\"id\":\"A\",\"label\":\"A\",\"type\":\"foundation.thermal.thermal\"},{\"id\":\"R\",\"label\":\"R\",\"type\":\"input\"}],\"Right\":[{\"id\":\"B\",\"label\":\"B\",\"type\":\"foundation.thermal.thermal\"}],\"Top\":[]}"
  Heat inlet : PMIOPort  Side=Left
  Heat exit : PMIOPort  Port=2  Side=Right
  wires:
  Relational Operator: Heating Switch/1 -> Memory/1
  T measurement/1 -> Relational Operator: Heating Switch/2
  High resistance: Off/1 -> Switch/3
  Switch/1 -> Scope/1, Simulink-PS Converter/1
  T target/1 -> Relational Operator: Heating Switch/1
  Memory/1 -> Logical Operator/2
  Logical Operator/1 -> Switch/2
  Low resistance: On/1 -> Switch/1
  Control Signal/1 -> Memory1/1
  Memory1/1 -> Logical Operator/1
  connections:
  Simulink-PS Converter/RConn1 -- Variable Thermal Resistance: Thermal Switch/LConn2
  Variable Thermal Resistance: Thermal Switch/LConn1 -- Heat inlet/RConn1
  Variable Thermal Resistance: Thermal Switch/RConn1 -- Heat exit/RConn1

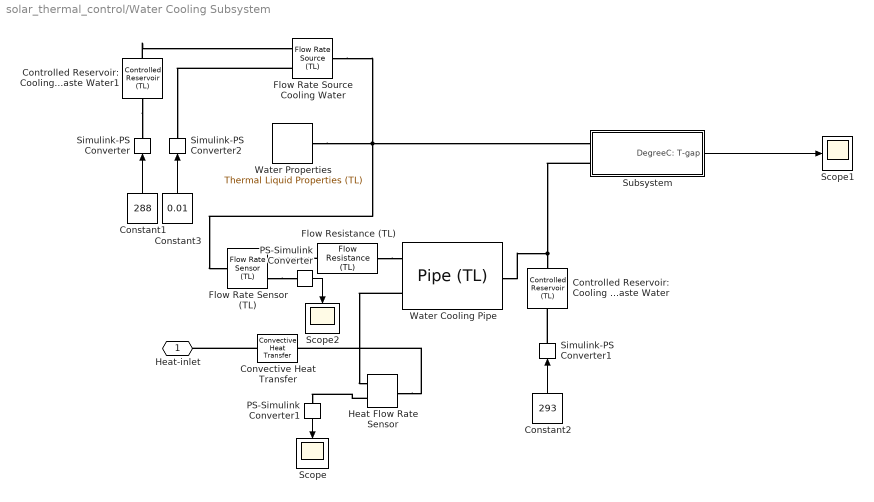
== system solar_thermal_control/Water Cooling Subsystem ==
  Constant1 : Constant  Value=288
  Constant2 : Constant  Value=293
  Constant3 : Constant  Value=0.01
  Controlled Reservoir: Cooling Waste Water : fl_lib/Thermal Liquid/Elements/Controlled Reservoir (TL)  pressure_spec=foundation.enum.pressure_spec.atmospheric  reservoir_pressure=0.101325 MPa  area=0.01 m^2
      settings: InternalSimscapePortConfiguration="{\"Bottom\":[],\"Left\":[{\"id\":\"A\",\"label\":\"A\",\"type\":\"foundation.thermal_liquid.thermal_liquid\"}],\"Right\":[{\"id\":\"T_in\",\"label\":\"T\",\"type\":\"input\"}],\"Top\":[]}"
  Controlled Reservoir: Cooling Waste Water1 : fl_lib/Thermal Liquid/Elements/Controlled Reservoir (TL)  pressure_spec=foundation.enum.pressure_spec.atmospheric  reservoir_pressure=0.101325 MPa  area=0.01 m^2
      settings: InternalSimscapePortConfiguration="{\"Bottom\":[],\"Left\":[{\"id\":\"A\",\"label\":\"A\",\"type\":\"foundation.thermal_liquid.thermal_liquid\"}],\"Right\":[{\"id\":\"T_in\",\"label\":\"T\",\"type\":\"input\"}],\"Top\":[]}"
  Convective Heat Transfer : fl_lib/Thermal/Thermal Elements/Convective Heat Transfer  thermal_type=foundation.enum.constant_variable.constant  area=0.1 m^2  heat_tr_coeff=150 W/(K*m^2)  min_heat_tr_coeff=1e-3 W/(K*m^2)  T_specify=off  T_priority=None  T=0 K  T_nominal_specify=off  T_nominal_value=1  T_nominal_unit=K  Q_specify=off  Q_priority=None  Q=0 W  Q_nominal_specify=off  Q_nominal_value=1  Q_nominal_unit=W
  Flow Rate Sensor (TL) : fl_lib/Thermal Liquid/Sensors/Flow Rate Sensor (TL)  mass_flow_measure=true  volumetric_flow_measure=false  energy_flow_measure=false
      settings: InternalSimscapePortConfiguration="{\"Bottom\":[],\"Left\":[{\"id\":\"A\",\"label\":\"A\",\"type\":\"foundation.thermal_liquid.thermal_liquid\"}],\"Right\":[{\"id\":\"B\",\"label\":\"B\",\"type\":\"foundation.thermal_liquid.thermal_liquid\"},{\"id\":\"M\",\"label\":\"M\",\"type\":\"output\"}],\"Top\":[]}"
  Flow Rate Source Cooling Water : fl_lib/Thermal Liquid/Sources/Flow Rate Source (TL)  source_type=foundation.enum.constant_controlled.controlled  flow_type=foundation.enum.mass_volumetric_flow.mass  mass_flow=0 kg/s  volumetric_flow=0 m^3/s  power_spec=foundation.enum.power_spec.isentropic  area=1e-4 m^2
  Flow Resistance (TL) : fl_lib/Thermal Liquid/Elements/Flow Resistance (TL)  delta_p_nominal=0.001 MPa  mdot_nominal=0.1 kg/s  area=1e-4 m^2  laminar_fraction=1e-3
  Heat Flow Rate Sensor : fl_lib/Thermal/Thermal Sensors/Heat Flow Rate Sensor
  PS-Simulink Converter : nesl_utility/PS-Simulink Converter  PhysicalDomain=network_engine_domain  SubClassName=ps_output  LeftPortType=input  RightPortType=output  PseudoPeriodic=off  Frequencies=[]  VectorFormat=inherit  Unit=inherit  AffineConversion=off
  PS-Simulink Converter1 : nesl_utility/PS-Simulink Converter  PhysicalDomain=network_engine_domain  SubClassName=ps_output  LeftPortType=input  RightPortType=output  PseudoPeriodic=off  Frequencies=[]  VectorFormat=inherit  Unit=inherit  AffineConversion=off
  Scope : Scope
  Scope1 : Scope
  Scope2 : Scope
  Simulink-PS Converter : nesl_utility/Simulink-PS Converter  PhysicalDomain=network_engine_domain  SubClassName=ps_input  LeftPortType=input  RightPortType=output  PseudoPeriodic=off  Frequencies=[]  NoiseDistribution=none  NoiseParameters=[]  Unit=1  AffineConversion=off  FilteringAndDerivatives=provide  SimscapeFilterOrder=1  InputFilterTimeConstant=0.001  UdotUserProvided=0
  Simulink-PS Converter1 : nesl_utility/Simulink-PS Converter  PhysicalDomain=network_engine_domain  SubClassName=ps_input  LeftPortType=input  RightPortType=output  PseudoPeriodic=off  Frequencies=[]  NoiseDistribution=none  NoiseParameters=[]  Unit=1  AffineConversion=off  FilteringAndDerivatives=provide  SimscapeFilterOrder=1  InputFilterTimeConstant=0.001  UdotUserProvided=0
  Simulink-PS Converter2 : nesl_utility/Simulink-PS Converter  PhysicalDomain=network_engine_domain  SubClassName=ps_input  LeftPortType=input  RightPortType=output  PseudoPeriodic=off  Frequencies=[]  NoiseDistribution=none  NoiseParameters=[]  Unit=1  AffineConversion=off  FilteringAndDerivatives=provide  SimscapeFilterOrder=1  InputFilterTimeConstant=0.001  UdotUserProvided=0
  Subsystem : Subsystem
  Water Properties : SimscapeFluids_lib/Thermal Liquid/Utilities/Thermal Liquid Properties (TL)  fluid_list=fluids.thermal_liquid.utilities.enum.thermal_liquid_fluid_list.water  concentration_param_EG=fluids.thermal_liquid.utilities.enum.thermal_liquid_concentration.volume_fraction  concentration_param_PG=fluids.thermal_liquid.utilities.enum.thermal_liquid_concentration.volume_fraction  c_mass_SW=3.5e-3  c_mass_EG=0.1  c_mass_PG=0.1  c_mass_GL=0.1  c_vol_EG=0.1  c_vol_PG=0.1  beta_const_EG=2.1791 GPa  beta_const_PG=2.1791 GPa  beta_const_GL=2.1791 GPa  p_min_EG=0.01 MPa  p_min_PG=0.01 MPa  p_min_GL=0.01 MPa  p_max_EG=50 MPa  p_max_PG=50 MPa  p_max_GL=50 MPa  p_atm=0.101325 MPa  properties_range_check=simscape.enum.assert.action.error
  Water Cooling Pipe : fl_lib/Thermal Liquid/Elements/Pipe (TL)  length=5 m  area=1e-4 m^2  Dh=0.1128 m  length_add=1 m  roughness=15e-6 m  Re_lam=2000  Re_tur=4000  shape_factor=64  Nu_lam=3.66  dynamic_compressibility=false  inertia=false  p0=0.101325 MPa  T0=293.15 K  mdot0=0 kg/s
  Heat-inlet : PMIOPort  Side=Left
  wires:
  Constant1/1 -> Simulink-PS Converter/1
  Subsystem/1(DegreeC: T-gap) -> Scope1/1
  PS-Simulink Converter/1 -> Scope2/1
  Constant2/1 -> Simulink-PS Converter1/1
  Constant3/1 -> Simulink-PS Converter2/1
  PS-Simulink Converter1/1 -> Scope/1
  connections:
  Simulink-PS Converter1/RConn1 -- Controlled Reservoir: Cooling Waste Water/RConn1
  Flow Resistance (TL)/LConn1 -- Flow Rate Sensor (TL)/RConn1
  Water Properties/RConn1 -- Subsystem/LConn1 -- Flow Rate Source Cooling Water/RConn1 -- Flow Rate Sensor (TL)/LConn1
  Water Cooling Pipe/RConn1 -- Subsystem/LConn2 -- Controlled Reservoir: Cooling Waste Water/LConn1
  Flow Resistance (TL)/RConn1 -- Water Cooling Pipe/LConn1
  Controlled Reservoir: Cooling Waste Water1/RConn1 -- Simulink-PS Converter/RConn1
  Controlled Reservoir: Cooling Waste Water1/LConn1 -- Flow Rate Source Cooling Water/LConn1
  Flow Rate Source Cooling Water/LConn2 -- Simulink-PS Converter2/RConn1
  Flow Rate Sensor (TL)/RConn2 -- PS-Simulink Converter/LConn1
  Water Cooling Pipe/LConn2 -- Heat Flow Rate Sensor/RConn2
  Heat Flow Rate Sensor/RConn1 -- PS-Simulink Converter1/LConn1
  Convective Heat Transfer/LConn1 -- Heat-inlet/RConn1
  Heat Flow Rate Sensor/LConn1 -- Convective Heat Transfer/RConn1

== system solar_thermal_control/Solar Thermal Source/DegreeC conversion ==
  Absolute zero reference : Constant  Value=-273.15
  PS-Simulink Converter : nesl_utility/PS-Simulink Converter  PhysicalDomain=network_engine_domain  SubClassName=ps_output  LeftPortType=input  RightPortType=output  PseudoPeriodic=off  Frequencies=[]  VectorFormat=inherit  Unit=inherit  AffineConversion=off
  T: degreeC : Sum
  PS-signal : PMIOPort  Side=Left
  DegreeC : Outport
  wires:
  Absolute zero reference/1 -> T: degreeC/2
  PS-Simulink Converter/1 -> T: degreeC/1
  T: degreeC/1 -> DegreeC/1
  connections:
  PS-signal/RConn1 -- PS-Simulink Converter/LConn1

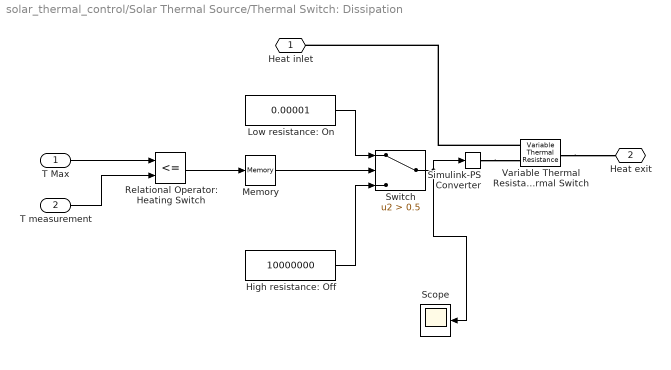
== system solar_thermal_control/Solar Thermal Source/Thermal Switch: Dissipation ==
  T Max : Inport
  T measurement : Inport  Port=2
  High resistance: Off : Constant  Value=10000000
  Low resistance: On : Constant  Value=0.00001
  Memory : Memory
  Relational Operator: Heating Switch : RelationalOperator  Operator=<=  OutDataTypeStr=boolean  RndMeth=Simplest  InputSameDT=off
  Scope : Scope
  Simulink-PS Converter : nesl_utility/Simulink-PS Converter  PhysicalDomain=network_engine_domain  SubClassName=ps_input  LeftPortType=input  RightPortType=output  PseudoPeriodic=off  Frequencies=[]  NoiseDistribution=none  NoiseParameters=[]  Unit=1  AffineConversion=off  FilteringAndDerivatives=provide  SimscapeFilterOrder=1  InputFilterTimeConstant=0.001  UdotUserProvided=0
  Switch : Switch  Criteria=u2 > Threshold  Threshold=0.5  SaturateOnIntegerOverflow=off  InputSameDT=off
  Variable Thermal Resistance: Thermal Switch : fl_lib/Thermal/Thermal Elements/Variable Thermal Resistance  R_min=0 K/W  T_specify=off  T_priority=None  T=0 K  T_nominal_specify=off  T_nominal_value=1  T_nominal_unit=K  Q_specify=off  Q_priority=None  Q=0 W  Q_nominal_specify=off  Q_nominal_value=1  Q_nominal_unit=W
      settings: InternalSimscapePortConfiguration="{\"Bottom\":[],\"Left\":[{\"id\":\"A\",\"label\":\"A\",\"type\":\"foundation.thermal.thermal\"},{\"id\":\"R\",\"label\":\"R\",\"type\":\"input\"}],\"Right\":[{\"id\":\"B\",\"label\":\"B\",\"type\":\"foundation.thermal.thermal\"}],\"Top\":[]}"
  Heat inlet : PMIOPort  Side=Left
  Heat exit : PMIOPort  Port=2  Side=Right
  wires:
  Relational Operator: Heating Switch/1 -> Memory/1
  T measurement/1 -> Relational Operator: Heating Switch/2
  High resistance: Off/1 -> Switch/3
  Switch/1 -> Scope/1, Simulink-PS Converter/1
  T Max/1 -> Relational Operator: Heating Switch/1
  Low resistance: On/1 -> Switch/1
  Memory/1 -> Switch/2
  connections:
  Simulink-PS Converter/RConn1 -- Variable Thermal Resistance: Thermal Switch/LConn2
  Variable Thermal Resistance: Thermal Switch/LConn1 -- Heat inlet/RConn1
  Variable Thermal Resistance: Thermal Switch/RConn1 -- Heat exit/RConn1

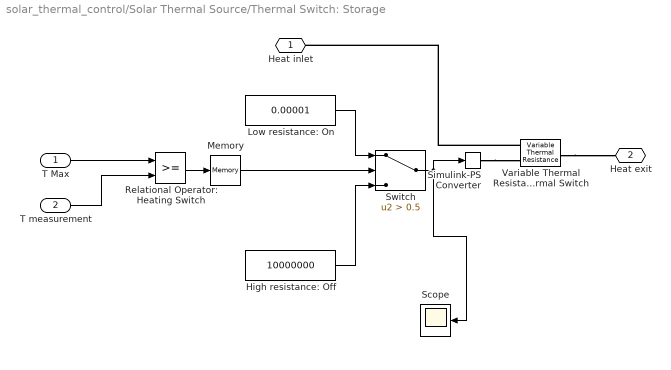
== system solar_thermal_control/Solar Thermal Source/Thermal Switch: Storage ==
  T Max : Inport
  T measurement : Inport  Port=2
  High resistance: Off : Constant  Value=10000000
  Low resistance: On : Constant  Value=0.00001
  Memory : Memory
  Relational Operator: Heating Switch : RelationalOperator  OutDataTypeStr=boolean  RndMeth=Simplest  InputSameDT=off
  Scope : Scope
  Simulink-PS Converter : nesl_utility/Simulink-PS Converter  PhysicalDomain=network_engine_domain  SubClassName=ps_input  LeftPortType=input  RightPortType=output  PseudoPeriodic=off  Frequencies=[]  NoiseDistribution=none  NoiseParameters=[]  Unit=1  AffineConversion=off  FilteringAndDerivatives=provide  SimscapeFilterOrder=1  InputFilterTimeConstant=0.001  UdotUserProvided=0
  Switch : Switch  Criteria=u2 > Threshold  Threshold=0.5  SaturateOnIntegerOverflow=off  InputSameDT=off
  Variable Thermal Resistance: Thermal Switch : fl_lib/Thermal/Thermal Elements/Variable Thermal Resistance  R_min=0 K/W  T_specify=off  T_priority=None  T=0 K  T_nominal_specify=off  T_nominal_value=1  T_nominal_unit=K  Q_specify=off  Q_priority=None  Q=0 W  Q_nominal_specify=off  Q_nominal_value=1  Q_nominal_unit=W
      settings: InternalSimscapePortConfiguration="{\"Bottom\":[],\"Left\":[{\"id\":\"A\",\"label\":\"A\",\"type\":\"foundation.thermal.thermal\"},{\"id\":\"R\",\"label\":\"R\",\"type\":\"input\"}],\"Right\":[{\"id\":\"B\",\"label\":\"B\",\"type\":\"foundation.thermal.thermal\"}],\"Top\":[]}"
  Heat inlet : PMIOPort  Side=Left
  Heat exit : PMIOPort  Port=2  Side=Right
  wires:
  Relational Operator: Heating Switch/1 -> Memory/1
  T measurement/1 -> Relational Operator: Heating Switch/2
  High resistance: Off/1 -> Switch/3
  Switch/1 -> Scope/1, Simulink-PS Converter/1
  T Max/1 -> Relational Operator: Heating Switch/1
  Low resistance: On/1 -> Switch/1
  Memory/1 -> Switch/2
  connections:
  Simulink-PS Converter/RConn1 -- Variable Thermal Resistance: Thermal Switch/LConn2
  Variable Thermal Resistance: Thermal Switch/LConn1 -- Heat inlet/RConn1
  Variable Thermal Resistance: Thermal Switch/RConn1 -- Heat exit/RConn1

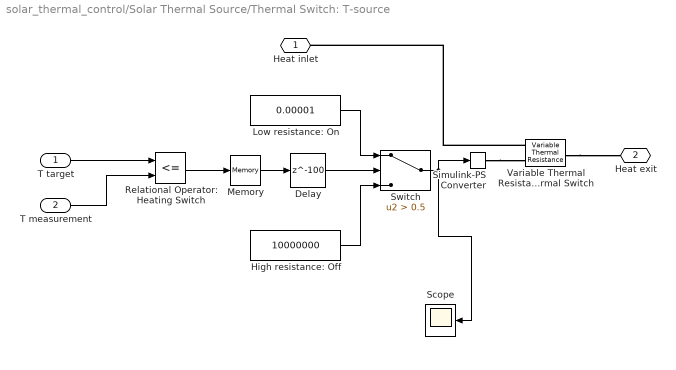
== system solar_thermal_control/Solar Thermal Source/Thermal Switch: T-source ==
  T target : Inport
  T measurement : Inport  Port=2
  Delay : Delay  DelayLength=100  InitialCondition=0
  High resistance: Off : Constant  Value=10000000
  Low resistance: On : Constant  Value=0.00001
  Memory : Memory
  Relational Operator: Heating Switch : RelationalOperator  Operator=<=  OutDataTypeStr=boolean  RndMeth=Simplest  InputSameDT=off
  Scope : Scope
  Simulink-PS Converter : nesl_utility/Simulink-PS Converter  PhysicalDomain=network_engine_domain  SubClassName=ps_input  LeftPortType=input  RightPortType=output  PseudoPeriodic=off  Frequencies=[]  NoiseDistribution=none  NoiseParameters=[]  Unit=1  AffineConversion=off  FilteringAndDerivatives=provide  SimscapeFilterOrder=1  InputFilterTimeConstant=0.001  UdotUserProvided=0
  Switch : Switch  Criteria=u2 > Threshold  Threshold=0.5  SaturateOnIntegerOverflow=off  InputSameDT=off
  Variable Thermal Resistance: Thermal Switch : fl_lib/Thermal/Thermal Elements/Variable Thermal Resistance  R_min=0 K/W  T_specify=off  T_priority=None  T=0 K  T_nominal_specify=off  T_nominal_value=1  T_nominal_unit=K  Q_specify=off  Q_priority=None  Q=0 W  Q_nominal_specify=off  Q_nominal_value=1  Q_nominal_unit=W
      settings: InternalSimscapePortConfiguration="{\"Bottom\":[],\"Left\":[{\"id\":\"A\",\"label\":\"A\",\"type\":\"foundation.thermal.thermal\"},{\"id\":\"R\",\"label\":\"R\",\"type\":\"input\"}],\"Right\":[{\"id\":\"B\",\"label\":\"B\",\"type\":\"foundation.thermal.thermal\"}],\"Top\":[]}"
  Heat inlet : PMIOPort  Side=Left
  Heat exit : PMIOPort  Port=2  Side=Right
  wires:
  Relational Operator: Heating Switch/1 -> Memory/1
  T measurement/1 -> Relational Operator: Heating Switch/2
  High resistance: Off/1 -> Switch/3
  Switch/1 -> Scope/1, Simulink-PS Converter/1
  T target/1 -> Relational Operator: Heating Switch/1
  Low resistance: On/1 -> Switch/1
  Memory/1 -> Delay/1
  Delay/1 -> Switch/2
  connections:
  Simulink-PS Converter/RConn1 -- Variable Thermal Resistance: Thermal Switch/LConn2
  Variable Thermal Resistance: Thermal Switch/LConn1 -- Heat inlet/RConn1
  Variable Thermal Resistance: Thermal Switch/RConn1 -- Heat exit/RConn1

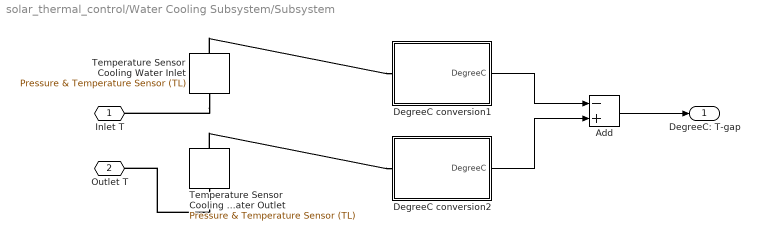
== system solar_thermal_control/Water Cooling Subsystem/Subsystem ==
  Add : Sum  Inputs=-+
  DegreeC conversion1 : Subsystem
  DegreeC conversion2 : Subsystem
  Temperature Sensor Cooling Water Inlet : fl_lib/Thermal Liquid/Sensors/Pressure & Temperature Sensor (TL)  reference=foundation.enum.MeasurementReference.absolute  pressure=false  pressure_spec=foundation.enum.PressureMeasementSpec.Absolute  temperature=true
      settings: InternalSimscapePortConfiguration="{\"Bottom\":[{\"id\":\"T\",\"label\":\"T\",\"type\":\"output\"}],\"Left\":[{\"id\":\"A\",\"label\":\"A\",\"type\":\"foundation.thermal_liquid.thermal_liquid\"}],\"Right\":[],\"Top\":[]}"
  Temperature Sensor Cooling Water Outlet : fl_lib/Thermal Liquid/Sensors/Pressure & Temperature Sensor (TL)  reference=foundation.enum.MeasurementReference.absolute  pressure=false  pressure_spec=foundation.enum.PressureMeasementSpec.Absolute  temperature=true
      settings: InternalSimscapePortConfiguration="{\"Bottom\":[{\"id\":\"T\",\"label\":\"T\",\"type\":\"output\"}],\"Left\":[{\"id\":\"A\",\"label\":\"A\",\"type\":\"foundation.thermal_liquid.thermal_liquid\"}],\"Right\":[],\"Top\":[]}"
  Inlet T : PMIOPort  Side=Left
  Outlet T : PMIOPort  Port=2  Side=Left
  DegreeC: T-gap : Outport
  wires:
  DegreeC conversion1/1(DegreeC) -> Add/1
  DegreeC conversion2/1(DegreeC) -> Add/2
  Add/1 -> DegreeC: T-gap/1
  connections:
  Temperature Sensor Cooling Water Outlet/RConn1 -- DegreeC conversion2/LConn1
  Temperature Sensor Cooling Water Inlet/RConn1 -- DegreeC conversion1/LConn1
  Temperature Sensor Cooling Water Outlet/LConn1 -- Outlet T/RConn1
  Temperature Sensor Cooling Water Inlet/LConn1 -- Inlet T/RConn1

== system solar_thermal_control/Water Cooling Subsystem/Subsystem/DegreeC conversion1 ==
  Absolute zero reference : Constant  Value=-273.15
  PS-Simulink Converter : nesl_utility/PS-Simulink Converter  PhysicalDomain=network_engine_domain  SubClassName=ps_output  LeftPortType=input  RightPortType=output  PseudoPeriodic=off  Frequencies=[]  VectorFormat=inherit  Unit=inherit  AffineConversion=off
  T: degreeC : Sum
  PS-signal : PMIOPort  Side=Left
  DegreeC : Outport
  wires:
  Absolute zero reference/1 -> T: degreeC/2
  PS-Simulink Converter/1 -> T: degreeC/1
  T: degreeC/1 -> DegreeC/1
  connections:
  PS-signal/RConn1 -- PS-Simulink Converter/LConn1

== system solar_thermal_control/Water Cooling Subsystem/Subsystem/DegreeC conversion2 ==
  Absolute zero reference : Constant  Value=-273.15
  PS-Simulink Converter : nesl_utility/PS-Simulink Converter  PhysicalDomain=network_engine_domain  SubClassName=ps_output  LeftPortType=input  RightPortType=output  PseudoPeriodic=off  Frequencies=[]  VectorFormat=inherit  Unit=inherit  AffineConversion=off
  T: degreeC : Sum
  PS-signal : PMIOPort  Side=Left
  DegreeC : Outport
  wires:
  Absolute zero reference/1 -> T: degreeC/2
  PS-Simulink Converter/1 -> T: degreeC/1
  T: degreeC/1 -> DegreeC/1
  connections:
  PS-signal/RConn1 -- PS-Simulink Converter/LConn1
